simulink library "commrandsrc2"  (Simulink 6.0)
settings: Solver=ode45  SolverMode=SingleTasking  StartTime=0.0  StopTime=10.0  RelTol=1e-3
libraries: dspsrcs4 x3, dspsigattribs x2, simulink x2
settings Model: Creator=akansal  LastModifiedBy=asuri
settings Model: ForwardingTableString=|
  | ||__slOldName__||commrandsrc2/Binary Error
  | Pattern Generator||__slNewName__||commnoisgen2/Binary Error
  | Pattern Generator
settings DataIOCC: SignalLoggingName=logsOut
settings OptimizationCC: BooleanDataType=off
settings DebuggingCC: CheckExecutionContextPreStartOutputMsg=on  CheckExecutionContextRuntimeOutputMsg=on  SolverPrmCheckMsg=none
settings HardwareCC: TargetUnknown=on
settings SFSimCC: SFSimApplyToAllLibs=on  SFSimBuildMode=Incremental

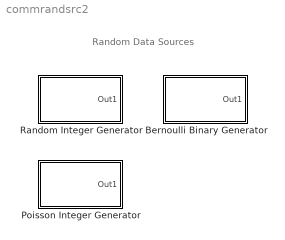
== system commrandsrc2 ==
  note: Random Data Sources
  Bernoulli Binary Generator : Subsystem  PropExecContextAcrossSSBoundary=on  mask(Bernoulli Binary Generator){P=0.5, seed=61, Ts=1, frameBased=off, sampPerFrame=1, orient=off}
      mask prompts: P "Probability of a zero:"; seed "Initial seed:"; Ts "Sample time:"; frameBased "Frame-based outputs"; sampPerFrame "Samples per frame:"; orient "Interpret vector parameters as 1-D"
      mask help:
      | Generate a Bernoulli random binary number.
      | To generate a vector output, specify the probability as a vector.
      mask init:
      | if (frameBased & sampPerFrame > 1)
      | 	dsp_sampFrame = sampPerFrame;
      | else
      | 	dsp_sampFrame = 1;
      | end;
      | [P, seed, eStr] = commblkbernoullisrc2(gcb,'init');
      | if (eStr.ecode == 1)
      |     error(eStr.emsg);
      | end;
      mask Help: helpview(commbhelp)
      mask CallbackString: |||commblkbernoullisrc2(gcb,'cbFrameBased');||commblkbernoullisrc2(gcb,'cbOrient');
      mask Display:
      | plot(0,0,100,100,[95 5 10 10 10 reshape(([85*[0:1/15:1-1/15]+10; 85*[1/15:1/15:1]+10]),1,30)],[75 75 75 70 95 90 90 90 90 80 80 80 80 90 90 80 80 80 80 90 90 90 90 80 80 80 80 90 90 90 90 80 80 90 90]);
      | disp('\nBernoulli\nBinary')
  Poisson Integer Generator : Subsystem  PropExecContextAcrossSSBoundary=on  mask(Poisson Integer Generator){lambda=0.1, seed=43, Ts=1, frameBased=off, sampPerFrame=1, orient=off}
      mask prompts: seed "Initial seed:"; Ts "Sample time:"; frameBased "Frame-based outputs"; sampPerFrame "Samples per frame:"; orient "Interpret vector parameters as 1-D"
      mask help: Generate Poisson distributed random integers.
      mask init:
      | [eStr, numChan, lambda, seed, orientSBVec] = commblkpoissrc(gcb, 'init');
      | if (eStr.ecode==1), 
      | 	error(eStr.emsg);
      | end;
      mask Help: helpview(commbhelp);
      mask CallbackString: |||commblkpoissrc(gcb,'cbFrameBased');||commblkpoissrc(gcb,'cbOrient');
      mask Display:
      | plot(0,0,100,100,[95 5 10 10 10 reshape(([85*[0:1/15:1-1/15]+10; 85*[1/15:1/15:1]+10]),1,30)],[75 75 75 70 95 reshape([randint(1,15,[75,95],54321); randint(1,15,[75,95],54321)],1,30)]);
      | disp('\nPoisson\nInteger');
  Random Integer Generator : Subsystem  PropExecContextAcrossSSBoundary=on  mask(Random Integer Generator){mul=8, seed=37, Ts=1, frameBased=off, sampPerFrame=1, orient=off}
      mask prompts: mul "M-ary number:"; seed "Initial seed:"; Ts "Sample time:"; frameBased "Frame-based outputs"; sampPerFrame "Samples per frame:"; orient "Interpret vector parameters as 1-D"
      mask help: Generate random uniformly distributed integers in the range [0, M-1], where M is the M-ary number.
      mask init:
      | if (frameBased & sampPerFrame > 1), dsp_sampFrame = sampPerFrame;
      | else dsp_sampFrame = 1; end
      | eStr=commblkrandintsrc2(gcb,'init');
      | if(eStr.ecode==1)
      |     error(eStr.emsg);
      | end
      mask Help: helpview(commbhelp)
      mask CallbackString: |||commblkrandintsrc2(gcb,'cbFrameBased');||commblkrandintsrc2(gcb,'cbOrient');
      mask Display:
      | plot(0,0,100,100,[95 5 10 10 10 reshape(([85*[0:1/15:1-1/15]+10; 85*[1/15:1/15:1]+10]),1,30)],[75 75 75 70 95 94 94 78 78 91 91 86 86 88 88 77 77 79 79 78 78 79 79 87 87 85 85 76 76 80 80 95 95 89 89]);
      | disp('\nRandom\nInteger')

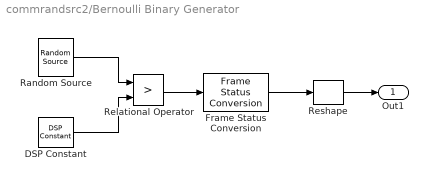
== system commrandsrc2/Bernoulli Binary Generator ==
  DSP Constant : dspsrcs4/DSP Constant  Value=P  SampleMode=Discrete  discreteOutput=Sample-based  continuousOutput=Sample-based  sampTime=Ts  framePeriod=Ts  dataType=Inherit from 'Constant value'  wordLen=16  udDataType=sfix(16)  fracBitsMode=Best precision  numFracBits=15  InterpretAs1D=off  Ts=Ts  FramebasedOutput=off
  Frame Status Conversion : dspsigattribs/Frame Status Conversion  growRefPort=off  outframe=Sample-based
  Random Source : dspsrcs4/Random Source  SrcType=Uniform  NormMethod=Ziggurat  CltLength=12  Min=0  Max=1  Mean=0  Var=1  RepMode=Specify seed  Seed=seed  Inherit=off  SampMode=Discrete  SampTime=Ts  SampFrame=dsp_sampFrame  DataType=Double  OutComplex=Real
  Relational Operator : RelationalOperator  Operator=>  LogicOutDataTypeMode=Specify via dialog  LogicDataType=float('double')  InputSameDT=on
  Reshape : simulink/Math Operations/Reshape  OutputDimensionality=Row vector  OutputDimensions=[sampPerFrame,max(length(P),length(seed))]
  Out1 : Outport
  wires:
  Frame Status Conversion/1 -> Reshape/1
  Reshape/1 -> Out1/1
  Relational Operator/1 -> Frame Status Conversion/1
  DSP Constant/1 -> Relational Operator/2
  Random Source/1 -> Relational Operator/1

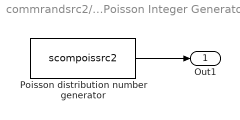
== system commrandsrc2/Poisson Integer Generator ==
  Poisson distribution number generator : S-Function  FunctionName=scompoissrc2  Parameters=seed, lambda, Ts, numChan, frameBased, sampPerFrame, orient, orientSBVec
  Out1 : Outport
  wires:
  Poisson distribution number generator/1 -> Out1/1

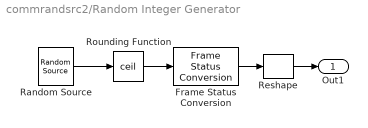
== system commrandsrc2/Random Integer Generator ==
  Frame Status Conversion : dspsigattribs/Frame Status Conversion  growRefPort=off  outframe=Sample-based
  Random Source : dspsrcs4/Random Source  SrcType=Uniform  NormMethod=Ziggurat  CltLength=12  Min=-1+eps  Max=mul-1  Mean=0  Var=1  RepMode=Specify seed  Seed=seed  Inherit=off  SampMode=Discrete  SampTime=Ts  SampFrame=dsp_sampFrame  DataType=Double  OutComplex=Real
  Reshape : simulink/Math Operations/Reshape  OutputDimensionality=Row vector  OutputDimensions=[sampPerFrame,max([length(mul), length(seed)])]
  Rounding Function : Rounding  Operator=ceil
  Out1 : Outport
  wires:
  Frame Status Conversion/1 -> Reshape/1
  Random Source/1 -> Rounding Function/1
  Reshape/1 -> Out1/1
  Rounding Function/1 -> Frame Status Conversion/1
